simulink model "SG2"  (R2013a)
settings: Solver=ode4  StartTime=0.0  StopTime=10.0  FixedStep=0.001  RelTol=1e-3
undefined symbols (not defined in the file): T_m
libraries: SG2_model x2
settings Model: Creator=USER  LastModifiedBy=USER

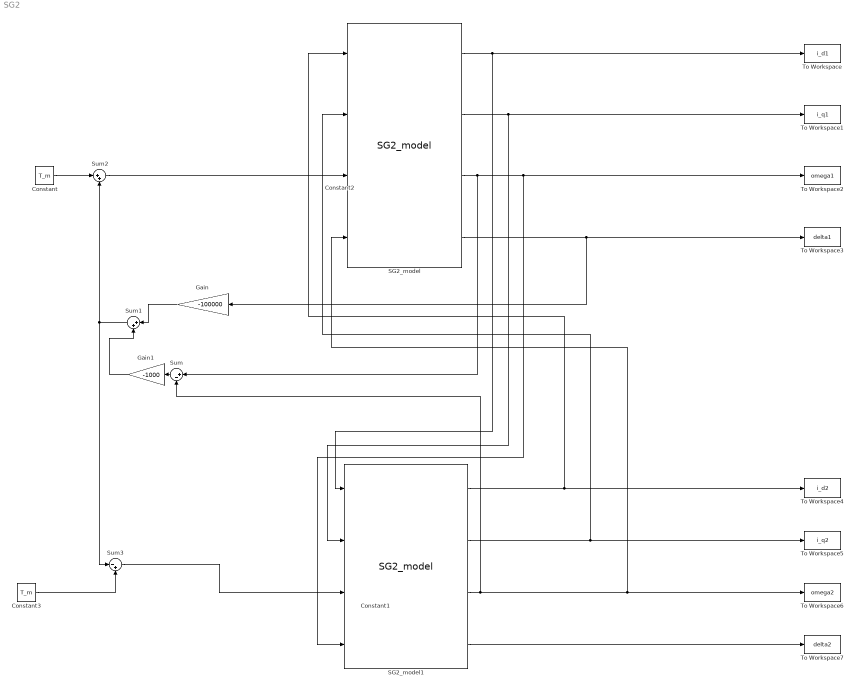
== system SG2 ==
  Constant{,1..3} (4 alike) : Constant  Value=T_m
  Gain : Gain  Gain=-100000
  Gain1 : Gain  Gain=-1000
  SG2_model : SG2_model/SG2_model  i_q0=i_q01  i_d0=i_d01  omega_0=omega_01  delta_0=delta_01
  SG2_model1 : SG2_model/SG2_model  i_q0=i_q02  i_d0=i_d02  omega_0=omega_02  delta_0=delta_02
  Sum : Sum  Inputs=|+-
  Sum1 : Sum  Inputs=|++
  Sum2 : Sum  Inputs=|++
  Sum3 : Sum  Inputs=|-+
  To Workspace : ToWorkspace  VariableName=i_d1  SampleTime=-1  SaveFormat=Timeseries
  To Workspace1 : ToWorkspace  VariableName=i_q1  SampleTime=-1  SaveFormat=Timeseries
  To Workspace2 : ToWorkspace  VariableName=omega1  SampleTime=-1  SaveFormat=Timeseries
  To Workspace3 : ToWorkspace  VariableName=delta1  SampleTime=-1  SaveFormat=Timeseries
  To Workspace4 : ToWorkspace  VariableName=i_d2  SampleTime=-1  SaveFormat=Timeseries
  To Workspace5 : ToWorkspace  VariableName=i_q2  SampleTime=-1  SaveFormat=Timeseries
  To Workspace6 : ToWorkspace  VariableName=omega2  SampleTime=-1  SaveFormat=Timeseries
  To Workspace7 : ToWorkspace  VariableName=delta2  SampleTime=-1  SaveFormat=Timeseries
  wires:
  SG2_model/1 -> SG2_model1/1, To Workspace/1
  SG2_model/2 -> To Workspace1/1, SG2_model1/2
  SG2_model/3 -> Sum/1, To Workspace2/1, SG2_model1/4
  SG2_model/4 -> Gain/1, To Workspace3/1
  SG2_model1/1 -> To Workspace4/1, SG2_model/1
  SG2_model1/2 -> SG2_model/2, To Workspace5/1
  SG2_model1/3 -> SG2_model/4, To Workspace6/1, Sum/2
  SG2_model1/4 -> To Workspace7/1
  Sum/1 -> Gain1/1
  Constant/1 -> Sum2/1
  Sum2/1 -> SG2_model/3
  Sum1/1 -> Sum2/2, Sum3/1
  Constant3/1 -> Sum3/2
  Sum3/1 -> SG2_model1/3
  Gain/1 -> Sum1/1
  Gain1/1 -> Sum1/2
